simulink model "COMH_Test"  (R2016a)
settings: Solver=VariableStepAuto  StartTime=0.0  StopTime=10.0  RelTol=1e-3
libraries: simulink x2, COMH x1
settings Model: Creator=oelkawok  LastModifiedBy=oelkawok

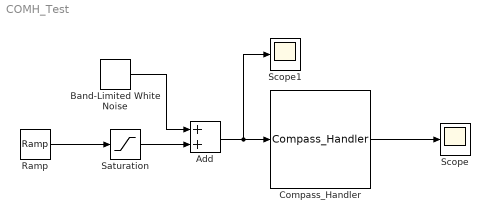
== system COMH_Test ==
  Add : Sum
  Band-Limited White Noise : simulink/Sources/Band-Limited White Noise  Cov=[0.1]  Ts=0.1  seed=[23341]
  Compass_Handler : COMH/Compass_Handler
  Ramp : simulink/Sources/Ramp  slope=40  start=0  X0=-10
  Saturation : Saturate  UpperLimit=380  LowerLimit=-10
  Scope : Scope
  Scope1 : Scope
  wires:
  Ramp/1 -> Saturation/1
  Saturation/1 -> Add/2
  Compass_Handler/1 -> Scope/1
  Band-Limited White Noise/1 -> Add/1
  Add/1 -> Scope1/1, Compass_Handler/1
